simulink model "blockdemo"  (Simulink 6.3)
settings: Solver=ode45  StartTime=0.0  StopTime=100  RelTol=1e-3
InitFcn:
  | %% DSPBuilder Start
  | alt_dspbuilder_update_model(bdroot)
  | %% DSPBuilder End
libraries: allblocks_alteradspbuilder2 x6
settings Model: Creator=cpurcell  LastModifiedBy=delphick
settings DebuggingCC: MultiTaskDSMMsg=error

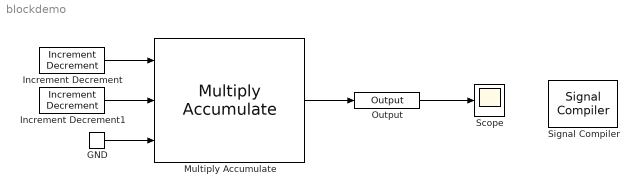
== system blockdemo ==
  GND : allblocks_alteradspbuilder2/GND  SpecifyClock=off
  Increment Decrement : allblocks_alteradspbuilder2/Increment Decrement  BusType=Signed Fractional  bwl=4  bwr=2  SpecifyClock=off  clr_value=0  direction=Increment  phase_selection=1  use_ena=off  use_sclr=off
  Increment Decrement1 : allblocks_alteradspbuilder2/Increment Decrement  BusType=Signed Fractional  bwl=4  bwr=2  SpecifyClock=off  clr_value=0  direction=Decrement  phase_selection=1  use_ena=off  use_sclr=off
  Multiply Accumulate : allblocks_alteradspbuilder2/Multiply Accumulate  BusType=Signed Fractional  abwl=4  abwr=2  bbwl=2  bbwr=4  ywidth=11  pipeline_register=Data Inputs and Multiplier  direction=Add  use_addsub=off  use_ena=off  use_aclr=off  UseDedicatedCircuitry=AUTO
  Output : allblocks_alteradspbuilder2/Output  iofile=C:\workspace_clean\Documentation\DesignExamples\Tutorials\UnitBlocks\Arithmetic\MultiplyAccumulate\tb_blockdemo\blockdemo_Output.capture  BusType=Inferred  bwl=8  bwr=0  PORTTYPE=Output
  Scope : Scope
      settings: TimeRange=100  YMin=-17  YMax=17
  Signal Compiler : allblocks_alteradspbuilder2/Signal Compiler  DeviceFamily=Stratix IV  DeviceName=AUTO  EnableSignalTap=off  SignalTapDepth=128  UseBoardBlock=off  StpUseDefaultClock=on  StpClock=clock
  wires:
  Increment Decrement/1 -> Multiply Accumulate/1
  Increment Decrement1/1 -> Multiply Accumulate/2
  GND/1 -> Multiply Accumulate/3
  Multiply Accumulate/1 -> Output/1
  Output/1 -> Scope/1
